simulink model "Cholesky_Ex2"  (R2025a)
settings: Solver=VariableStepAuto  StartTime=0.0  StopTime=10  RelTol=1e-3
InitFcn:
  | A = single(rand(8,8));
undefined symbols (not defined in the file): S, static_input_Convolution_Stream_Ex1, Subsystem, vsva2197, xcvc1902
libraries: aieSolver x1, aieUtilities x1, vmcUtilities x1
settings Model: Creator=sdegala  LastModifiedBy=sdegala
settings ModelReferenceCC: EnableRefExpFcnMdlSchedulingChecks=on
settings RTWCC: GPUComputeCapability=3.5

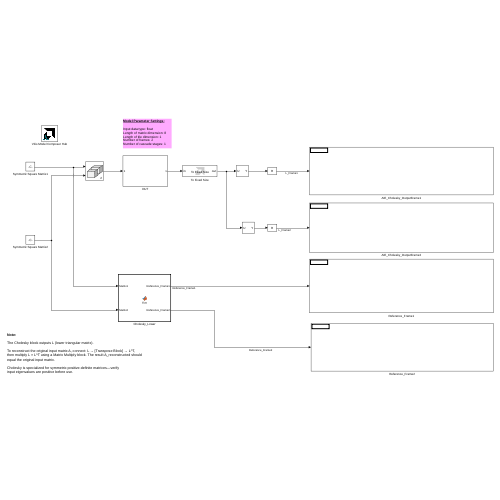
[thumbnail: Simulink's stored preview of the top-level diagram]
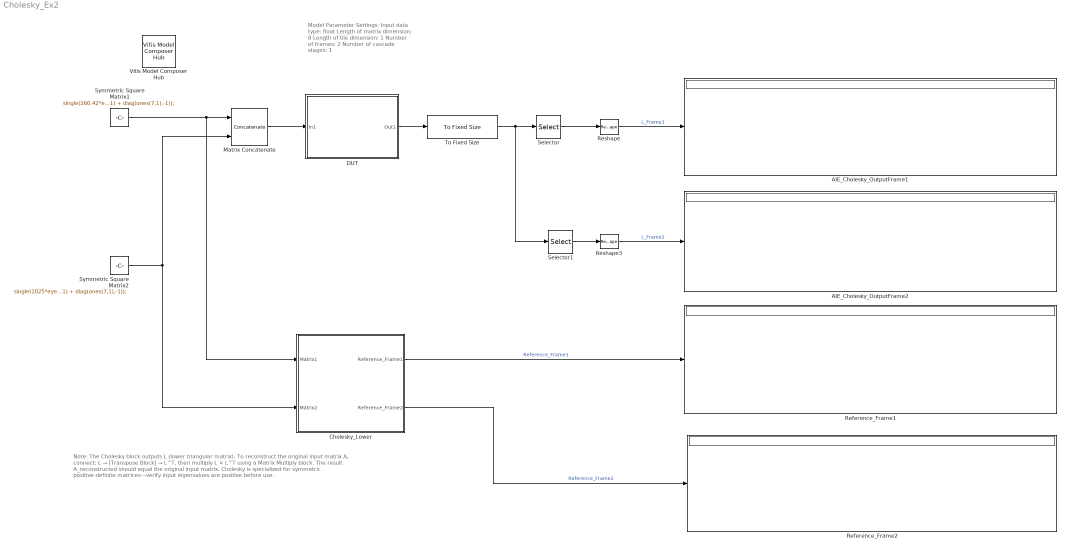
== system Cholesky_Ex2 ==
  note: Model Parameter Settings:
      |
      | Input data type: float
      | Length of matrix dimension: 8
      | Length of tile dimension: 1
      | Number of frames: 2
      | Number of cascade stages: 1
  note: Note:
      |
      | The Cholesky block outputs L (lower triangular matrix).
      |
      | To reconstruct the original input matrix A, connect: L → [Transpose Block] → L^T,
      | then multiply L × L^T using a Matrix Multiply block. The result A_reconstructed should
      | equal the original input matrix.
      |
      | Cholesky is specialized for symmetric positive-definite matrices—verify
      | input eigenvalues are positive before use.
  AIE_Cholesky_OutputFrame1 : Display
  AIE_Cholesky_OutputFrame2 : Display
  Cholesky_Lower : MATLAB Function  TreatAsAtomicUnit=on
  DUT : Subsystem
  Matrix Concatenate : Concatenate  Mode=Multidimensional array  ConcatenateDimension=2
  Reference_Frame1 : Display
  Reference_Frame2 : Display
  Reshape : Reshape  OutputDimensionality=Customize  OutputDimensions=[8,8]
  Reshape3 : Reshape  OutputDimensionality=Customize  OutputDimensions=[8,8]
  Selector : Selector  InputPortWidth=128  IndexOptions=Index vector (dialog)  Indices=1:64  OutputSizes=1
  Selector1 : Selector  InputPortWidth=128  IndexOptions=Index vector (dialog)  Indices=65:128  OutputSizes=1
  Symmetric Square Matrix1 : Constant  Value=single(260.42*eye(8) + diag(ones(7,1),1) + diag(ones(7,1),-1));  OutDataTypeStr=single  SampleTime=1
  Symmetric Square Matrix2 : Constant  Value=single(1025*eye(8) + diag(ones(7,1),1) + diag(ones(7,1),-1));  OutDataTypeStr=single  SampleTime=1
  To Fixed Size : aieUtilities/To Fixed Size  Mode=Stop simulation when input variable-size signal is not full  OutputSize=Inherit: Same as input  CopyMethod=Buffer samples to form output  HasStatusOutput=on
  Vitis Model Composer Hub : vmcUtilities/Vitis Model Composer Hub  Tag=genX  CodeGeneration=off  SubsystemName=Subsystem  BlockHierPath=static_input_Convolution_Stream_Ex1/Subsystem  SubsystemType=AIENode  AIEArrayConfig=Use entire AIE array  StartColumn=1  NumberOfColumns=1  TargetDirectory=./code  exportDesign=on  analyzeDesign=off  validateDesignOnHw=off  ExportType=AI Engines  IpVendor=xilinx.com  IpLibrary=hls  IpVersion=1.0  IpHWLanguage=Verilog  AieCompilerOptions={}  AieSimulatorOptions={}  CreateTestbench=on  TestbenchStackSize=10  RunRtlSim=off  RunCSim=off  RunAieSim=off  enableSimulationTimeout=on  enableGraphIterations=on  AieSimTimeout=50000  AieGraphIterations=-1  RunAieSimProfiling=off  LaunchVitisAnalyzer=off  PlotOutput=off  RunX86Sim=off  X86SimTimeout=10  GenHwImage=off  GenLibadfXo=off  GenHwValidationCode=off  PlatformType=Not Specified  HwSystemType=Baremetal  HwValidationTarget=hw  ProjDevice=xcvc1902-vsva2197-1LP-e-S  ProjDevicePart=xcvc1902-vsva2197-1LP-e-S  AIEType=AIE  SamplePeriod=-1  ClockFrequency=200  DataPathParallelism=1  xilinxfamily=versalaicore  part=xcvc1902  speed=-1LP-e-S  package=vsva2197  directory=./netlist  testbench=off  incr_netlist=off  synthesis_tool=Vivado  clock_wrapper=Clock Enables  dbl_ovrd=According to Block Masks  dcm_input_clock_period=10  sysclk_period=10  simulink_period=1  eval_field=0  IPInfoJsonString="{\"DUTSubsystemName\":\"Subsystem\",\"AIESubsystem\":{\"SubsystemName\":\"Subsystem\",\"TargetDirectory\":\"./code\",\"AIEArrayConfig\":\"Use entire AIE array\",\"StartColumn\":\"0\",\"NumberOfColumns\":\"1\"},\"SubsystemTag\":\"AIENode\"}"  LogFileName=/tmp/CR-1250814/code/model_composer.log  NThreads=4  IPConfigFile=/tmp/vmctmp-13380004059271250980/static_input_Convolution_Stream_Ex1_ipconfig.json
  wires:
  To Fixed Size/1 -> Selector1/1, Selector/1
  Cholesky_Lower/1(Reference_Frame1) -> Reference_Frame1/1  "Reference_Frame1"
  Reshape/1 -> AIE_Cholesky_OutputFrame1/1  "L_Frame1"
  DUT/1(Out1) -> To Fixed Size/1
  Symmetric Square Matrix2/1 -> Matrix Concatenate/2, Cholesky_Lower/2(Matrix2)
  Selector/1 -> Reshape/1
  Selector1/1 -> Reshape3/1
  Reshape3/1 -> AIE_Cholesky_OutputFrame2/1  "L_Frame2"
  Symmetric Square Matrix1/1 -> Cholesky_Lower/1(Matrix1), Matrix Concatenate/1
  Cholesky_Lower/2(Reference_Frame2) -> Reference_Frame2/1  "Reference_Frame2"
  Matrix Concatenate/1 -> DUT/1(In1)

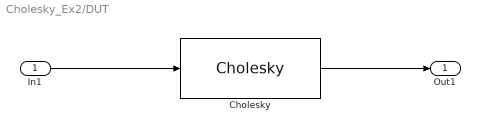
== system Cholesky_Ex2/DUT ==
  In1 : Inport
  Cholesky : aieSolver/Cholesky  AIE_VARIANT=1  data_type=float  dim_matrix=8  grid_dimension=1  num_frames=2  casc_length=1  inversion_diag=off  blockJsonConstraints=[]  blockJsonConstraintsInternal=[]  spec=vmc_cholesky.json  SerializedMaskParamNames=[]  SerializedMaskParamValues=[]  SerializedMaskParamVisibilities=[]  block_type=Cholesky  SerializedMaskParamDataypes=uint|typename|uint|uint|uint|uint|uint  SerializedMaskParamEnumStrArr=0|0|0|0|0|0|0  SerializedMaskParamEnumValArr=0|0|0|0|0|0|0  SerializedMaskParamVectorArr=0|0|0|0|0|0|0  SerializedMaskParamKeys=AIE_VARIANT|TT_DATA|TP_DIM|TP_GRID_DIM|TP_NUM_FRAMES|TP_CASC_LEN|TP_DIAG_INV
  Out1 : Outport
  wires:
  Cholesky/1 -> Out1/1
  In1/1 -> Cholesky/1

== matlab function Cholesky_Ex2/Cholesky_Lower ==
  data: Matrix1 input; Reference_Frame1 output; Matrix2 input; Reference_Frame2 output
function [Reference_Frame1,Reference_Frame2] = fcn(Matrix1,Matrix2)

Reference_Frame1 = single(chol(Matrix1,'lower'));

Reference_Frame2 = single(chol(Matrix2,'lower'));
